simulink model "Actuator"  (R2023a)
settings: Solver=VariableStepAuto  StartTime=0.0  StopTime=10.0  RelTol=1e-3
undefined symbols (not defined in the file or in its folder): motor_wm
settings Model: Creator=Tan_Tram  LastModifiedBy=Tan_Tram

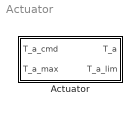
== system Actuator ==
  Actuator : Subsystem

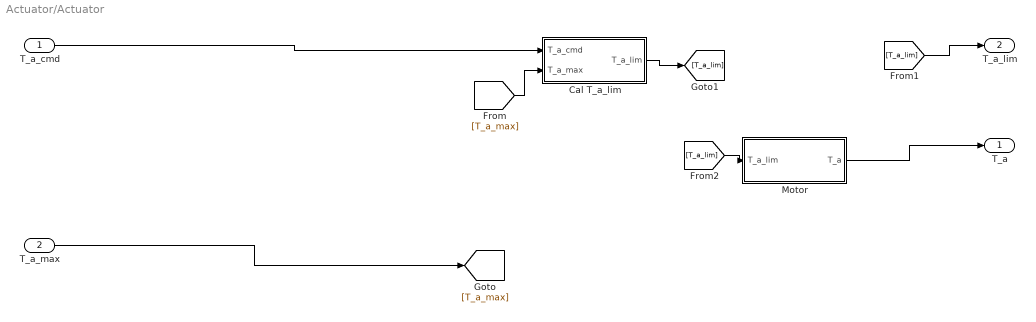
== system Actuator/Actuator ==
  T_a_cmd : Inport
  T_a_max : Inport  Port=2
  Cal T_a_lim : Subsystem
  Motor : Subsystem
  T_a : Outport
  T_a_lim : Outport  Port=2
  wires:
  T_a_max/1 -> [T_a_max]
  T_a_cmd/1 -> Cal T_a_lim/1(T_a_cmd)
  [T_a_max] -> Cal T_a_lim/2(T_a_max)
  Cal T_a_lim/1(T_a_lim) -> [T_a_lim]
  [T_a_lim] -> T_a_lim/1
  [T_a_lim] -> Motor/1(T_a_lim)
  Motor/1(T_a) -> T_a/1

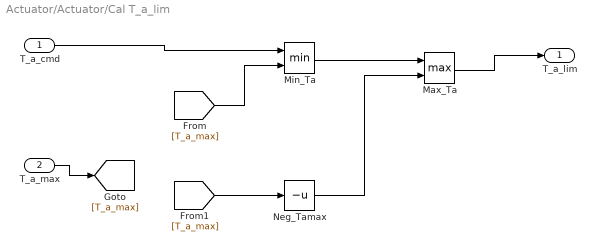
== system Actuator/Actuator/Cal T_a_lim ==
  T_a_cmd : Inport
  T_a_max : Inport  Port=2
  Max_Ta : MinMax  Function=max  Inputs=2
  Min_Ta : MinMax  Inputs=2
  Neg_Tamax : UnaryMinus
  T_a_lim : Outport
  wires:
  T_a_max/1 -> [T_a_max]
  T_a_cmd/1 -> Min_Ta/1
  [T_a_max] -> Min_Ta/2
  [T_a_max] -> Neg_Tamax/1
  Min_Ta/1 -> Max_Ta/1
  Neg_Tamax/1 -> Max_Ta/2
  Max_Ta/1 -> T_a_lim/1

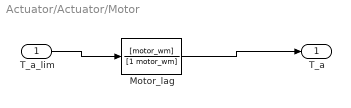
== system Actuator/Actuator/Motor ==
  T_a_lim : Inport
  Motor_lag : TransferFcn  Numerator=[motor_wm]  Denominator=[1 motor_wm]
  T_a : Outport
  wires:
  T_a_lim/1 -> Motor_lag/1
  Motor_lag/1 -> T_a/1
